simulink model "cukModelStateSpace"  (R2020a)
settings: Solver=FixedStepAuto  StartTime=0.0  StopTime=0.8  RelTol=1e-9  AbsTol=4e-3
undefined symbols (not defined in the file): Asigma, bsigma, Csigma, delta, FaultTypeArray, fdiDevices, fmaxArray, fminArray, Fsigma, Msigma, Nsigma, tfArray, x0, z0
libraries: PhdLibrary x7, powerlib_meascontrol x1
settings Model: SimulationMode=accelerator  Creator=d13go  LastModifiedBy=d13go
settings SolverCC: ZeroCrossControl=DisableAll  ZeroCrossAlgorithm=Adaptive
settings DebuggingCC: IgnoredZcDiagnostic=none

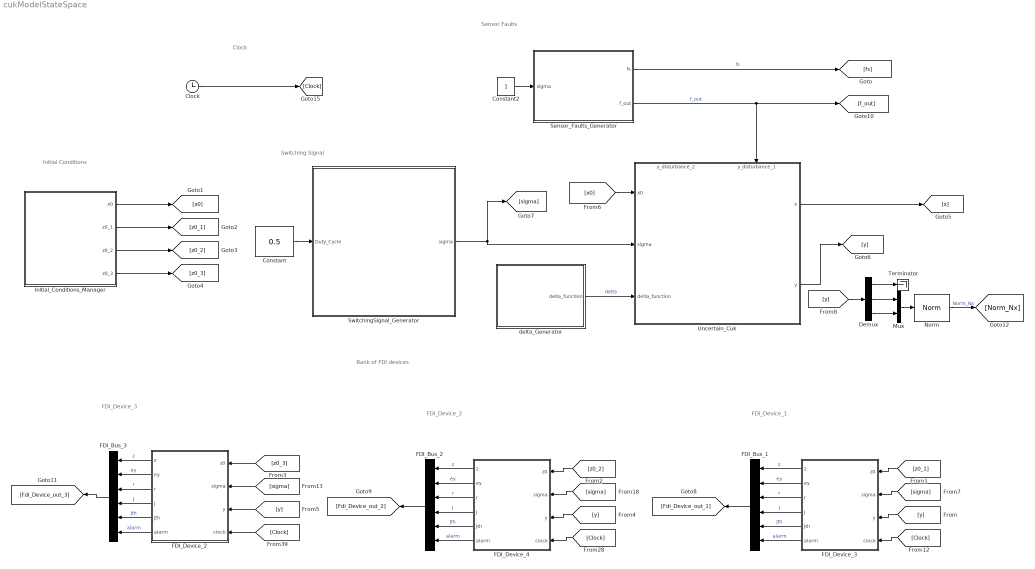
== system cukModelStateSpace ==
  note: Initial Condiitons
  note: Bank of FDI devices
  note: Sensor Faults
  note: FDI_Device_1
  note: FDI_Device_2
  note: FDI_Device_3
  note: Switching Signal
  note: Clock
  Clock : Clock
  Constant : Constant  Value=0.5
  Constant2 : Constant
  Demux : Demux  Outputs=3
  "FDI_Bus_1 " : BusCreator  Inputs=6
  FDI_Bus_2 : BusCreator  Inputs=6
  FDI_Bus_3 : BusCreator  Inputs=6
  FDI_Device_2 : Subsystem  mask{fdiDevice=fdiDevices{3}}
      mask prompts: fdiDevice "FDI Device (Struct)"
      mask Display: fprintf('FDI Device \n Two subsystems');
  FDI_Device_3 : Subsystem  mask{fdiDevice=fdiDevices{1}}
      mask prompts: fdiDevice "FDI Device (Struct)"
      mask Display: fprintf('FDI Device \n Two subsystems');
  FDI_Device_4 : Subsystem  mask{fdiDevice=fdiDevices{2}}
      mask prompts: fdiDevice "FDI Device (Struct)"
      mask Display: fprintf('FDI Device \n Two subsystems');
  Initial_Conditions_Manager : Subsystem
  Mux : Mux  Inputs=2
  Norm : PhdLibrary/Norms/Norm
      settings: SourceProductName=Phd Diego
  Sensor_Faults_Generator : Subsystem
  SwitchingSignal_Generator : Subsystem
  Terminator : Terminator
  Uncertain_Cuk : Subsystem
      settings: PortSchema="{\"entries\":[{\"content\":{\"sides\":[{\"content\":{\"connectorIds\":[\"In1\",\"In2\",\"In3\"]},\"type\":\"ConnectorPlacement.EquallySpacedRectSide\",\"uuid\":\"603634da-9cb1-4386-a493-85de7a0b3601\"},{\"content\":{\"connectorIds\":[\"Out1\",\"Out2\"],\"side\":\"RIGHT\"},\"type\":\"ConnectorPlacement.EquallySpacedRectSide\",\"uuid\":\"04120757-a7c7-4ef9-83e5-a164762aa976\"},{\"content\":{\"connectorIds\":[\"In4\",\"In5\"],\"side\":\"TOP\"},\"type\":\"ConnectorPlacement.EquallySpacedRectSide\",\"uuid\":\"e5c3024c-3e8e-4670-bb80-bfeaf8b64197\"}]},\"type\":\"ConnectorPlacement.EquallySpacedConnector\",\"uuid\":\"63699195-fae3-40a4-a348-448298818555\"}],\"packageUris\":[\"http://schema.mathworks.com/mf0/Connector/19700101\"],\"version\":\"1.0\"}"
  delta_Generator : Subsystem
  wires:
  Clock/1 -> [Clock]
  Sensor_Faults_Generator/2(f_out) -> Uncertain_Cuk/5(y_disturbance_1), [f_out]  "f_out"
  Constant2/1 -> Sensor_Faults_Generator/1(sigma)
  Sensor_Faults_Generator/1(fs) -> [fs]  "fs"
  Initial_Conditions_Manager/1(x0) -> [x0]
  Initial_Conditions_Manager/2(z0_1) -> [z0_1]
  Initial_Conditions_Manager/4(z0_3) -> [z0_3]
  Initial_Conditions_Manager/3(z0_2) -> [z0_2]
  [y] -> FDI_Device_3/3(y)
  [y] -> FDI_Device_4/3(y)
  [y] -> FDI_Device_2/3(y)
  SwitchingSignal_Generator/1(sigma) -> Uncertain_Cuk/2(sigma), [sigma]
  [sigma] -> FDI_Device_3/2(sigma)
  [sigma] -> FDI_Device_4/2(sigma)
  [sigma] -> FDI_Device_2/2(sigma)
  [Clock] -> FDI_Device_3/4(clock)
  [Clock] -> FDI_Device_4/4(clock)
  [Clock] -> FDI_Device_2/4(clock)
  [z0_2] -> FDI_Device_4/1(z0)
  [z0_3] -> FDI_Device_2/1(z0)
  delta_Generator/1(delta_function) -> Uncertain_Cuk/3(delta_function)  "delta"
  Constant/1 -> SwitchingSignal_Generator/1(Duty_Cycle)
  FDI_Device_3/1(z) -> "FDI_Bus_1 "/1  "z"
  FDI_Device_3/2(ey) -> "FDI_Bus_1 "/2  "ey"
  FDI_Device_3/3(r) -> "FDI_Bus_1 "/3  "r"
  FDI_Device_3/4(J) -> "FDI_Bus_1 "/4  "J"
  FDI_Device_4/1(z) -> FDI_Bus_2/1  "z"
  FDI_Device_4/2(ey) -> FDI_Bus_2/2  "ey"
  FDI_Device_4/3(r) -> FDI_Bus_2/3  "r"
  FDI_Device_4/4(J) -> FDI_Bus_2/4  "J"
  FDI_Device_2/1(z) -> FDI_Bus_3/1  "z"
  FDI_Device_2/2(ey) -> FDI_Bus_3/2  "ey"
  FDI_Device_2/3(r) -> FDI_Bus_3/3  "r"
  FDI_Device_2/4(J) -> FDI_Bus_3/4  "J"
  "FDI_Bus_1 "/1 -> [Fdi_Device_out_1]
  FDI_Bus_2/1 -> [Fdi_Device_out_2]
  FDI_Bus_3/1 -> [Fdi_Device_out_3]
  [z0_1] -> FDI_Device_3/1(z0)
  FDI_Device_3/5(Jth) -> "FDI_Bus_1 "/5  "Jth"
  FDI_Device_3/6(alarm) -> "FDI_Bus_1 "/6  "alarm"
  FDI_Device_4/5(Jth) -> FDI_Bus_2/5  "Jth"
  FDI_Device_4/6(alarm) -> FDI_Bus_2/6  "alarm"
  FDI_Device_2/5(Jth) -> FDI_Bus_3/5  "Jth"
  FDI_Device_2/6(alarm) -> FDI_Bus_3/6  "alarm"
  [x0] -> Uncertain_Cuk/1(x0)
  Uncertain_Cuk/2(y) -> [y]
  Uncertain_Cuk/1(x) -> [x]
  ? -> Uncertain_Cuk/4(y_disturbance_2)
  [y] -> Demux/1
  Demux/1 -> Terminator/1
  Mux/1 -> Norm/1
  Norm/1 -> [Norm_Nx]  "Norm_Nx"
  Demux/2 -> Mux/1
  Demux/3 -> Mux/2

== system cukModelStateSpace/FDI_Device_2 ==
  z0 : Inport  PortDimensions=4
  sigma : Inport  Port=2
  y : Inport  Port=3  PortDimensions=3
  clock : Inport  Port=4
  Alarm_Function : Subsystem
  Constant : Constant  Value=fdiDevice.Jth
  Resiual_Evaluation_Function : Subsystem
  Switched Residual Generator2 : Subsystem  AncestorBlock=PhdLibrary/Observers/Switched Residual Generator  mask(Boots State-Space model){reg_z=fdiDevice.regs_z}
      mask prompts: reg_z "Residual error generator (struct)"
      mask help: Boots State-Space model
      mask DialogControl DescTextVar Prompt: dxhat/dt = A(sigma)*xhat+B(sigma)*u + L(sigma)*(y-yhat)
      mask DialogControl Control2 Prompt: yhat = C(sigma)*xhat
      mask DialogControl Control3 Prompt: r = R(sigma)*(y-yhat)
      mask DialogControl Subsystem1 Prompt: Subsystem 1
      mask Display: disp('Switched Luenberger \n Residual Generator \n 2-Subsystems')
  Terminator : Terminator
  z : Outport
  ey : Outport  Port=2
  r : Outport  Port=3
  J : Outport  Port=4
  Jth : Outport  Port=5
  alarm : Outport  Port=6
  wires:
  sigma/1 -> Switched Residual Generator2/2(sigma)
  Alarm_Function/1(alarm) -> alarm/1
  Switched Residual Generator2/4(ey) -> ey/1
  [r] -> r/1
  clock/1 -> [clock]
  [clock] -> Resiual_Evaluation_Function/2(clock)
  Resiual_Evaluation_Function/1(J) -> J/1, Alarm_Function/1(J)
  Switched Residual Generator2/3(r) -> [r], Resiual_Evaluation_Function/1(r)
  Constant/1 -> Jth/1, Alarm_Function/2(Jth)
  y/1 -> Switched Residual Generator2/3(y)
  Switched Residual Generator2/1(z) -> z/1
  z0/1 -> Switched Residual Generator2/1(x0)
  Switched Residual Generator2/2(yhat) -> Terminator/1

== system cukModelStateSpace/FDI_Device_3 ==
  z0 : Inport  PortDimensions=4
  sigma : Inport  Port=2
  y : Inport  Port=3  PortDimensions=3
  clock : Inport  Port=4
  Alarm_Function : Subsystem
  Constant : Constant  Value=fdiDevice.Jth
  Resiual_Evaluation_Function : Subsystem
  Switched Residual Generator2 : Subsystem  AncestorBlock=PhdLibrary/Observers/Switched Residual Generator  mask(Boots State-Space model){reg_z=fdiDevice.regs_z}
      mask prompts: reg_z "Residual error generator (struct)"
      mask help: Boots State-Space model
      mask DialogControl DescTextVar Prompt: dxhat/dt = A(sigma)*xhat+B(sigma)*u + L(sigma)*(y-yhat)
      mask DialogControl Control2 Prompt: yhat = C(sigma)*xhat
      mask DialogControl Control3 Prompt: r = R(sigma)*(y-yhat)
      mask DialogControl Subsystem1 Prompt: Subsystem 1
      mask Display: disp('Switched Luenberger \n Residual Generator \n 2-Subsystems')
  Terminator : Terminator
  z : Outport
  ey : Outport  Port=2
  r : Outport  Port=3
  J : Outport  Port=4
  Jth : Outport  Port=5
  alarm : Outport  Port=6
  wires:
  sigma/1 -> Switched Residual Generator2/2(sigma)
  Alarm_Function/1(alarm) -> alarm/1
  Switched Residual Generator2/4(ey) -> ey/1
  [r] -> r/1
  clock/1 -> [clock]
  [clock] -> Resiual_Evaluation_Function/2(clock)
  Resiual_Evaluation_Function/1(J) -> J/1, Alarm_Function/1(J)
  Switched Residual Generator2/3(r) -> [r], Resiual_Evaluation_Function/1(r)
  Constant/1 -> Jth/1, Alarm_Function/2(Jth)
  y/1 -> Switched Residual Generator2/3(y)
  Switched Residual Generator2/1(z) -> z/1
  z0/1 -> Switched Residual Generator2/1(x0)
  Switched Residual Generator2/2(yhat) -> Terminator/1

== system cukModelStateSpace/FDI_Device_4 ==
  z0 : Inport  PortDimensions=4
  sigma : Inport  Port=2
  y : Inport  Port=3  PortDimensions=3
  clock : Inport  Port=4
  Alarm_Function : Subsystem
  Constant : Constant  Value=fdiDevice.Jth
  Resiual_Evaluation_Function1 : Subsystem
  Switched Residual Generator2 : Subsystem  AncestorBlock=PhdLibrary/Observers/Switched Residual Generator  mask(Boots State-Space model){reg_z=fdiDevice.regs_z}
      mask prompts: reg_z "Residual error generator (struct)"
      mask help: Boots State-Space model
      mask DialogControl DescTextVar Prompt: dxhat/dt = A(sigma)*xhat+B(sigma)*u + L(sigma)*(y-yhat)
      mask DialogControl Control2 Prompt: yhat = C(sigma)*xhat
      mask DialogControl Control3 Prompt: r = R(sigma)*(y-yhat)
      mask DialogControl Subsystem1 Prompt: Subsystem 1
      mask Display: disp('Switched Luenberger \n Residual Generator \n 2-Subsystems')
  Terminator : Terminator
  z : Outport
  ey : Outport  Port=2
  r : Outport  Port=3
  J : Outport  Port=4
  Jth : Outport  Port=5
  alarm : Outport  Port=6
  wires:
  sigma/1 -> Switched Residual Generator2/2(sigma)
  Alarm_Function/1(alarm) -> alarm/1
  Switched Residual Generator2/4(ey) -> ey/1
  [r] -> r/1
  clock/1 -> [clock]
  [clock] -> Resiual_Evaluation_Function1/2(clock)
  Resiual_Evaluation_Function1/1(J) -> J/1, Alarm_Function/1(J)
  Switched Residual Generator2/3(r) -> Resiual_Evaluation_Function1/1(r), [r]
  Constant/1 -> Jth/1, Alarm_Function/2(Jth)
  y/1 -> Switched Residual Generator2/3(y)
  Switched Residual Generator2/1(z) -> z/1
  z0/1 -> Switched Residual Generator2/1(x0)
  Switched Residual Generator2/2(yhat) -> Terminator/1

== system cukModelStateSpace/Initial_Conditions_Manager ==
  Ground1 : Ground
  IC1 : InitialCondition  Value=[x0]
  IC2 : InitialCondition  Value=[z0]
  Mux2 : Mux
  x0 : Outport
  z0_1 : Outport  Port=2
  z0_2 : Outport  Port=3
  z0_3 : Outport  Port=4
  wires:
  Mux2/1 -> IC1/1, IC2/1
  Ground1/1 -> Mux2/3, Mux2/4, Mux2/2, Mux2/1
  IC1/1 -> z0_1/1, x0/1
  IC2/1 -> z0_3/1, z0_2/1

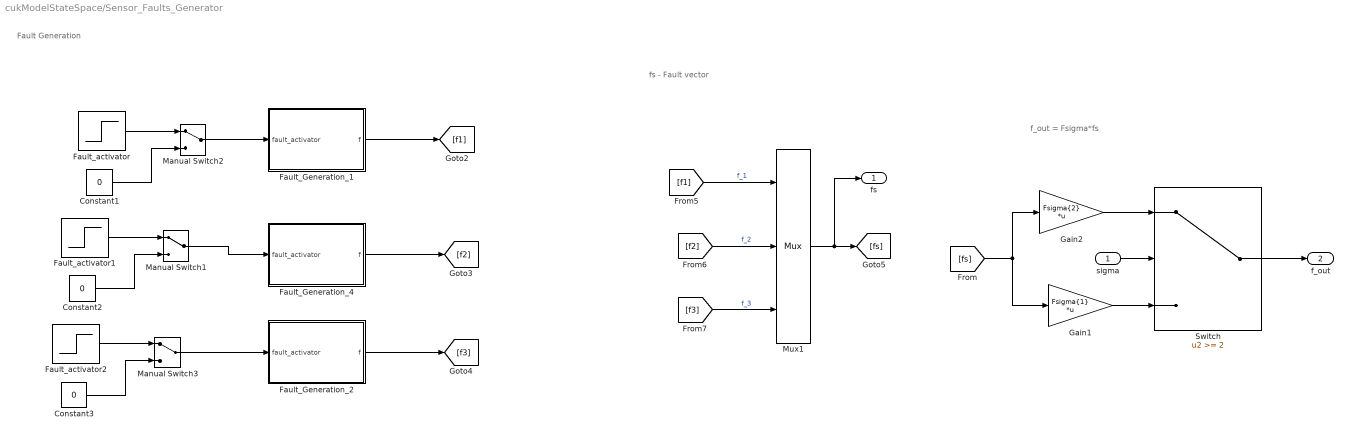
== system cukModelStateSpace/Sensor_Faults_Generator ==
  note: fs - Fault vector
  note: Fault Generation
  note: f_out = Fsigma*fs
  sigma : Inport
  Constant1 : Constant  Value=0
  Constant2 : Constant  Value=0
  Constant3 : Constant  Value=0
  Fault_Generation_1 : Subsystem  mask{fmax=fmaxArray(1), fmin=fminArray(1)}
      mask prompts: fmax "Maximum magnitude of the fault"; fmin "Minimum magnitude of the fault"
      mask DialogControl DescTextVar Prompt: Offset fatul generator.
      mask DialogControl DescTextVar_copy Prompt: Fault_activator:  0: f = 0; 1: f = fmax;  2  f =fmin
      mask Display: fprintf('Offset fault generator \n with two levels')
  Fault_Generation_2 : Subsystem  mask{fmax=fmaxArray(3), fmin=fminArray(3)}
      mask prompts: fmax "Maximum magnitude of the fault"; fmin "Minimum magnitude of the fault"
      mask DialogControl DescTextVar Prompt: Offset fatul generator.
      mask DialogControl DescTextVar_copy Prompt: Fault_activator:  0: f = 0; 1: f = fmax;  2  f =fmin
      mask Display: fprintf('Offset fault generator \n with two levels')
  Fault_Generation_4 : Subsystem  mask{fmax=fmaxArray(2), fmin=fminArray(2)}
      mask prompts: fmax "Maximum magnitude of the fault"; fmin "Minimum magnitude of the fault"
      mask DialogControl DescTextVar Prompt: Offset fatul generator.
      mask DialogControl DescTextVar_copy Prompt: Fault_activator:  0: f = 0; 1: f = fmax;  2  f =fmin
      mask Display: fprintf('Offset fault generator \n with two levels')
  Fault_activator : Step  Time=tfArray(1)  After=FaultTypeArray(1)  SampleTime=0
  Fault_activator1 : Step  Time=tfArray(2)  After=FaultTypeArray(2)  SampleTime=0
  Fault_activator2 : Step  Time=tfArray(3)  After=FaultTypeArray(3)  SampleTime=0
  Gain1 : Gain  Gain=Fsigma{1}  Multiplication=Matrix(K*u) (u vector)
  Gain2 : Gain  Gain=Fsigma{2}  Multiplication=Matrix(K*u) (u vector)
  Manual Switch1 : ManualSwitch
  Manual Switch2 : ManualSwitch
  Manual Switch3 : ManualSwitch
  Mux1 : Mux  Inputs=3
      settings: DisplayOption=signals
  Switch : Switch  Threshold=2
  fs : Outport
  f_out : Outport  Port=2
  wires:
  Fault_Generation_4/1(f) -> [f2]
  [f1] -> Mux1/1  "f_1"
  [f2] -> Mux1/2  "f_2"
  [f3] -> Mux1/3  "f_3"
  Mux1/1 -> fs/1, [fs]
  sigma/1 -> Switch/2
  Gain1/1 -> Switch/3
  [fs] -> Gain2/1, Gain1/1
  Fault_Generation_1/1(f) -> [f1]
  Constant1/1 -> Manual Switch2/2
  Fault_activator/1 -> Manual Switch2/1
  Manual Switch2/1 -> Fault_Generation_1/1(fault_activator)
  Manual Switch1/1 -> Fault_Generation_4/1(fault_activator)
  Fault_activator1/1 -> Manual Switch1/1
  Constant2/1 -> Manual Switch1/2
  Manual Switch3/1 -> Fault_Generation_2/1(fault_activator)
  Fault_activator2/1 -> Manual Switch3/1
  Constant3/1 -> Manual Switch3/2
  Fault_Generation_2/1(f) -> [f3]
  Switch/1 -> f_out/1
  Gain2/1 -> Switch/1

== system cukModelStateSpace/SwitchingSignal_Generator ==
  Duty_Cycle : Inport
  Constant : Constant  Value=2
  PWM Generator (DC-DC)1 : powerlib_meascontrol/Pulse & Signal Generators/PWM Generator (DC-DC)  Fsw=20000  Ts=0
  Sum : Sum  Inputs=|-+
  sigma : Outport
  wires:
  Duty_Cycle/1 -> PWM Generator (DC-DC)1/1
  Constant/1 -> Sum/2
  PWM Generator (DC-DC)1/1 -> Sum/1
  Sum/1 -> sigma/1

== system cukModelStateSpace/Uncertain_Cuk ==
  x0 : Inport  PortDimensions=4
  sigma : Inport  Port=2
  delta_function : Inport  Port=3
  y_disturbance_2 : Inport  Port=4  PortDimensions=3
  y_disturbance_1 : Inport  Port=5  PortDimensions=3
  Uncertain Cuk : Subsystem  mask{A1=Asigma{1}, B1=bsigma{1}, C1=Csigma{1}, A2=Asigma{2}, B2=bsigma{2}, C2=Csigma{2}}
      mask prompts: A1 "Matrix A"; B1 "Matrix B"; C1 "Matrix C"; A2 "Matrix A"; B2 "Matrix B"; C2 "Matrix C"
      mask DialogControl DescTextVar Prompt: dx/dt = A(sigma)x+ b(sigma) + wx(sigma,x,u,t)
      mask DialogControl Control2 Prompt: y = C(sigma)x + wy(sigma,x,u,t)
      mask DialogControl Container3 Prompt: Subsystem 1
      mask DialogControl Container4 Prompt: Subsystem 2
      mask Display: disp('Switched Affine System State Space  \n with perturbations \n 2-Subsystems')
  Uncertainty_System_1 : Subsystem  mask{M=Msigma{1}, N=Nsigma{1}}
      mask prompts: M "M matrix"; N "N matrix"
      mask DialogControl DescTextVar Prompt: Uncertainties matrices of type \DeltaA = delta(t)*MaNa*x(t)
      mask Display: disp('Norm-bounded \n uncertainty')
  Uncertainty_System_2 : Subsystem  mask{M=Msigma{2}, N=Nsigma{2}}
      mask prompts: M "M matrix"; N "N matrix"
      mask DialogControl DescTextVar Prompt: Uncertainties matrices of type \DeltaA = delta(t)*MaNa*x(t)
      mask Display: disp('Norm-bounded \n uncertainty')
  x : Outport
  y : Outport  Port=2
  wires:
  [x] -> Uncertainty_System_2/2(x), Uncertainty_System_1/2(x)
  Uncertainty_System_2/1(DeltaAx) -> [DeltaA2x]
  Uncertain Cuk/1(x) -> x/1, [x]
  Uncertain Cuk/2(y) -> y/1
  delta_function/1 -> Uncertainty_System_1/1(delta_function), Uncertainty_System_2/1(delta_function)
  sigma/1 -> Uncertain Cuk/2(sigma)
  x0/1 -> Uncertain Cuk/1(x0)
  [DeltaA2x] -> Uncertain Cuk/5(x_disturbance_2)
  [DeltaA1x] -> Uncertain Cuk/3(x_disturbance_1)
  y_disturbance_2/1 -> Uncertain Cuk/6(y_disturbance_2)
  y_disturbance_1/1 -> Uncertain Cuk/4(y_disturbance_1)
  Uncertainty_System_1/1(DeltaAx) -> [DeltaA1x]

== system cukModelStateSpace/delta_Generator ==
  Constant : Constant  Value=0
  Manual Switch : ManualSwitch
  Sinusoidal : SignalGenerator  Amplitude=delta  Frequency=60  Units=rad/sec
  delta_function : Outport
  wires:
  Sinusoidal/1 -> Manual Switch/1
  Manual Switch/1 -> [delta], delta_function/1
  Constant/1 -> Manual Switch/2

== system cukModelStateSpace/FDI_Device_2/Alarm_Function ==
  note: If J(r)>=Jth, then a fault has occurred
  J : Inport
  Jth : Inport  Port=2
  Cast To Double : DataTypeConversion  OutDataTypeStr=double
  Constant : Constant
  Constant1 : Constant  Value=0
  GreaterThan : RelationalOperator  OutDataTypeStr=boolean  RndMeth=Simplest
  If : If
  If Action Subsystem : Subsystem  TreatAsAtomicUnit=on
  If Action Subsystem1 : Subsystem  TreatAsAtomicUnit=on
  Merge : Merge
  alarm : Outport
  wires:
  J/1 -> GreaterThan/1
  Jth/1 -> GreaterThan/2
  If/1 -> If Action Subsystem/Action
  Constant/1 -> If Action Subsystem/1(In1)
  If/2 -> If Action Subsystem1/Action
  Constant1/1 -> If Action Subsystem1/1(In1)
  If Action Subsystem/1(Out1) -> Merge/1
  If Action Subsystem1/1(Out1) -> Merge/2
  Merge/1 -> alarm/1
  GreaterThan/1 -> Cast To Double/1
  Cast To Double/1 -> If/1

== system cukModelStateSpace/FDI_Device_2/Resiual_Evaluation_Function ==
  r : Inport
  clock : Inport  Port=2
  Delay : Delay  DelayLength=1  SampleTime=fdiDevice.T
  If : If  IfExpression=u1 >= T
  If Action Subsystem : Subsystem  TreatAsAtomicUnit=on
  If Action Subsystem1 : Subsystem  TreatAsAtomicUnit=on
  Max : MinMax  Function=max  Inputs=2
  Merge : Merge
  Norm3 : PhdLibrary/Norms/Norm
      settings: SourceProductName=Phd Diego
  J : Outport
  wires:
  clock/1 -> If/1
  If/1 -> If Action Subsystem/Action
  If/2 -> If Action Subsystem1/Action
  r/1 -> [r]
  [r] -> Norm3/1
  [r] -> If Action Subsystem1/1(r)
  If Action Subsystem/1(J) -> Merge/1
  If Action Subsystem1/1(J) -> Merge/2
  Merge/1 -> J/1
  Delay/1 -> Max/2
  Norm3/1 -> Max/1, Delay/1  "||r1||"
  Max/1 -> If Action Subsystem/1(r)

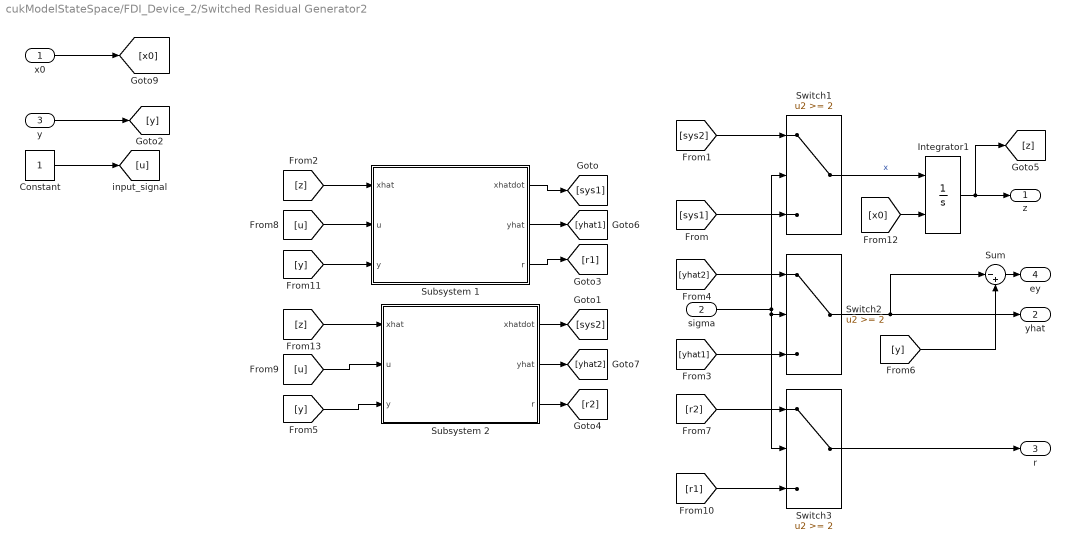
== system cukModelStateSpace/FDI_Device_2/Switched Residual Generator2 ==
  x0 : Inport
  sigma : Inport  Port=2
  y : Inport  Port=3
  Constant : Constant
  Integrator1 : Integrator  InitialConditionSource=external  InitialCondition=[0; 0; 0;0]
  Subsystem 1 : Subsystem  mask{A=reg_z.Asigma{1}, B=reg_z.bsigma{1}, L=reg_z.Lsigma{1}, C=reg_z.Csigma{1}, R=reg_z.Rsigma{1}}
      mask prompts: A "Matrix A"; B "Matrix B"; L "Matrix L"; C "Matrix C"; R "Matrix R"
      mask DialogControl DescTextVar Prompt: dxhat/dt = A*xhat + B*u + L*(y-yhat)
      mask DialogControl Control2 Prompt: yhat = C*xhat
      mask Display: disp('Luenberger Residual \n Generator')
  Subsystem 2 : Subsystem  mask{A=reg_z.Asigma{2}, B=reg_z.bsigma{2}, L=reg_z.Lsigma{2}, C=reg_z.Csigma{2}, R=reg_z.Rsigma{2}}
      mask prompts: A "Matrix A"; B "Matrix B"; L "Matrix L"; C "Matrix C"; R "Matrix R"
      mask DialogControl DescTextVar Prompt: dxhat/dt = A*xhat + B*u + L*(y-yhat)
      mask DialogControl Control2 Prompt: yhat = C*xhat
      mask Display: disp('Luenberger Residual \n Generator')
  Sum : Sum  Inputs=|-+
  Switch1 : Switch  Threshold=2
  Switch2 : Switch  Threshold=2
  Switch3 : Switch  Threshold=2
  z : Outport
  yhat : Outport  Port=2
  r : Outport  Port=3
  ey : Outport  Port=4
  wires:
  [yhat2] -> Switch2/1
  [yhat1] -> Switch2/3
  [y] -> Sum/2
  Sum/1 -> ey/1
  y/1 -> [y]
  [y] -> Subsystem 2/3(y)
  Switch3/1 -> r/1
  Switch2/1 -> yhat/1, Sum/1
  [r1] -> Switch3/3
  [r2] -> Switch3/1
  Subsystem 2/2(yhat) -> [yhat2]
  Subsystem 1/2(yhat) -> [yhat1]
  Subsystem 2/3(r) -> [r2]
  Subsystem 1/3(r) -> [r1]
  Subsystem 2/1(xhatdot) -> [sys2]
  Subsystem 1/1(xhatdot) -> [sys1]
  x0/1 -> [x0]
  Switch1/1 -> Integrator1/1  "x"
  [sys1] -> Switch1/3
  [sys2] -> Switch1/1
  Integrator1/1 -> [z], z/1
  sigma/1 -> Switch1/2, Switch2/2, Switch3/2
  Constant/1 -> [u]
  [u] -> Subsystem 1/2(u)
  [u] -> Subsystem 2/2(u)
  [y] -> Subsystem 1/3(y)
  [z] -> Subsystem 1/1(xhat)
  [z] -> Subsystem 2/1(xhat)
  [x0] -> Integrator1/2

== system cukModelStateSpace/FDI_Device_3/Alarm_Function ==
  note: If J(r)>=Jth, then a fault has occurred
  J : Inport
  Jth : Inport  Port=2
  Cast To Double : DataTypeConversion  OutDataTypeStr=double
  Constant : Constant
  Constant1 : Constant  Value=0
  GreaterThan : RelationalOperator  OutDataTypeStr=boolean  RndMeth=Simplest
  If : If
  If Action Subsystem : Subsystem  TreatAsAtomicUnit=on
  If Action Subsystem1 : Subsystem  TreatAsAtomicUnit=on
  Merge : Merge
  alarm : Outport
  wires:
  J/1 -> GreaterThan/1
  Jth/1 -> GreaterThan/2
  If/1 -> If Action Subsystem/Action
  Constant/1 -> If Action Subsystem/1(In1)
  If/2 -> If Action Subsystem1/Action
  Constant1/1 -> If Action Subsystem1/1(In1)
  If Action Subsystem/1(Out1) -> Merge/1
  If Action Subsystem1/1(Out1) -> Merge/2
  Merge/1 -> alarm/1
  GreaterThan/1 -> Cast To Double/1
  Cast To Double/1 -> If/1

== system cukModelStateSpace/FDI_Device_3/Resiual_Evaluation_Function ==
  r : Inport
  clock : Inport  Port=2
  Delay : Delay  DelayLength=1  SampleTime=fdiDevice.T
  If : If  IfExpression=u1 >= T
  If Action Subsystem : Subsystem  TreatAsAtomicUnit=on
  If Action Subsystem1 : Subsystem  TreatAsAtomicUnit=on
  Max : MinMax  Function=max  Inputs=2
  Merge : Merge
  Norm3 : PhdLibrary/Norms/Norm
      settings: SourceProductName=Phd Diego
  J : Outport
  wires:
  clock/1 -> If/1
  If/1 -> If Action Subsystem/Action
  If/2 -> If Action Subsystem1/Action
  r/1 -> [r]
  [r] -> Norm3/1
  [r] -> If Action Subsystem1/1(r)
  If Action Subsystem/1(J) -> Merge/1
  If Action Subsystem1/1(J) -> Merge/2
  Merge/1 -> J/1
  Delay/1 -> Max/2
  Norm3/1 -> Max/1, Delay/1  "||r1||"
  Max/1 -> If Action Subsystem/1(r)

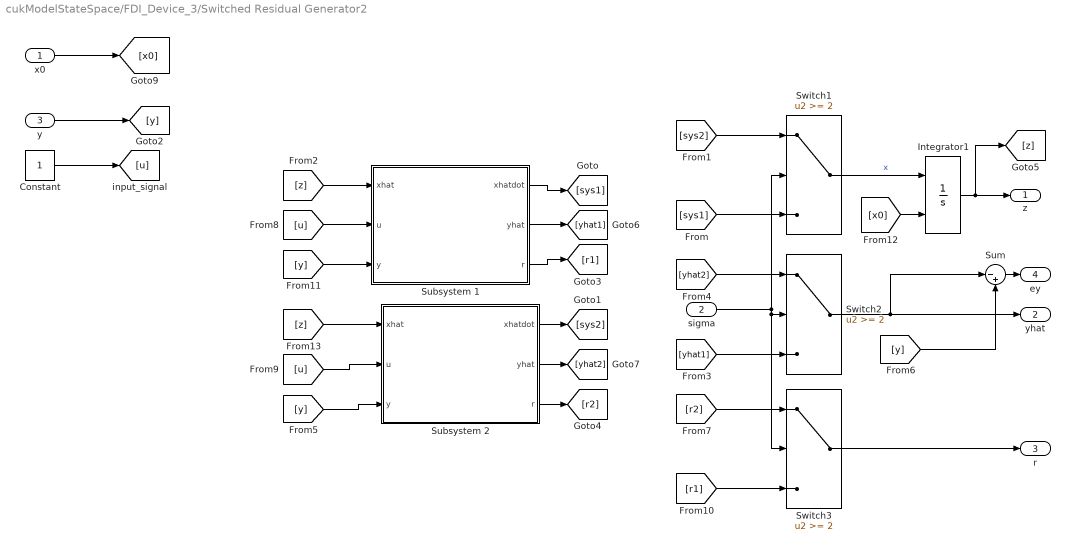
== system cukModelStateSpace/FDI_Device_3/Switched Residual Generator2 ==
  x0 : Inport
  sigma : Inport  Port=2
  y : Inport  Port=3
  Constant : Constant
  Integrator1 : Integrator  InitialConditionSource=external  InitialCondition=[0; 0; 0;0]
  Subsystem 1 : Subsystem  mask{A=reg_z.Asigma{1}, B=reg_z.bsigma{1}, L=reg_z.Lsigma{1}, C=reg_z.Csigma{1}, R=reg_z.Rsigma{1}}
      mask prompts: A "Matrix A"; B "Matrix B"; L "Matrix L"; C "Matrix C"; R "Matrix R"
      mask DialogControl DescTextVar Prompt: dxhat/dt = A*xhat + B*u + L*(y-yhat)
      mask DialogControl Control2 Prompt: yhat = C*xhat
      mask Display: disp('Luenberger Residual \n Generator')
  Subsystem 2 : Subsystem  mask{A=reg_z.Asigma{2}, B=reg_z.bsigma{2}, L=reg_z.Lsigma{2}, C=reg_z.Csigma{2}, R=reg_z.Rsigma{2}}
      mask prompts: A "Matrix A"; B "Matrix B"; L "Matrix L"; C "Matrix C"; R "Matrix R"
      mask DialogControl DescTextVar Prompt: dxhat/dt = A*xhat + B*u + L*(y-yhat)
      mask DialogControl Control2 Prompt: yhat = C*xhat
      mask Display: disp('Luenberger Residual \n Generator')
  Sum : Sum  Inputs=|-+
  Switch1 : Switch  Threshold=2
  Switch2 : Switch  Threshold=2
  Switch3 : Switch  Threshold=2
  z : Outport
  yhat : Outport  Port=2
  r : Outport  Port=3
  ey : Outport  Port=4
  wires:
  [yhat2] -> Switch2/1
  [yhat1] -> Switch2/3
  [y] -> Sum/2
  Sum/1 -> ey/1
  y/1 -> [y]
  [y] -> Subsystem 2/3(y)
  Switch3/1 -> r/1
  Switch2/1 -> yhat/1, Sum/1
  [r1] -> Switch3/3
  [r2] -> Switch3/1
  Subsystem 2/2(yhat) -> [yhat2]
  Subsystem 1/2(yhat) -> [yhat1]
  Subsystem 2/3(r) -> [r2]
  Subsystem 1/3(r) -> [r1]
  Subsystem 2/1(xhatdot) -> [sys2]
  Subsystem 1/1(xhatdot) -> [sys1]
  x0/1 -> [x0]
  Switch1/1 -> Integrator1/1  "x"
  [sys1] -> Switch1/3
  [sys2] -> Switch1/1
  Integrator1/1 -> [z], z/1
  sigma/1 -> Switch1/2, Switch2/2, Switch3/2
  Constant/1 -> [u]
  [u] -> Subsystem 1/2(u)
  [u] -> Subsystem 2/2(u)
  [y] -> Subsystem 1/3(y)
  [z] -> Subsystem 1/1(xhat)
  [z] -> Subsystem 2/1(xhat)
  [x0] -> Integrator1/2

== system cukModelStateSpace/FDI_Device_4/Alarm_Function ==
  note: If J(r)>=Jth, then a fault has occurred
  J : Inport
  Jth : Inport  Port=2
  Cast To Double : DataTypeConversion  OutDataTypeStr=double
  Constant : Constant
  Constant1 : Constant  Value=0
  GreaterThan : RelationalOperator  OutDataTypeStr=boolean  RndMeth=Simplest
  If : If
  If Action Subsystem : Subsystem  TreatAsAtomicUnit=on
  If Action Subsystem1 : Subsystem  TreatAsAtomicUnit=on
  Merge : Merge
  alarm : Outport
  wires:
  J/1 -> GreaterThan/1
  Jth/1 -> GreaterThan/2
  If/1 -> If Action Subsystem/Action
  Constant/1 -> If Action Subsystem/1(In1)
  If/2 -> If Action Subsystem1/Action
  Constant1/1 -> If Action Subsystem1/1(In1)
  If Action Subsystem/1(Out1) -> Merge/1
  If Action Subsystem1/1(Out1) -> Merge/2
  Merge/1 -> alarm/1
  GreaterThan/1 -> Cast To Double/1
  Cast To Double/1 -> If/1

== system cukModelStateSpace/FDI_Device_4/Resiual_Evaluation_Function1 ==
  r : Inport
  clock : Inport  Port=2
  Delay : Delay  DelayLength=1  SampleTime=fdiDevice.T
  If : If  IfExpression=u1 >= T
  If Action Subsystem : Subsystem  TreatAsAtomicUnit=on
  If Action Subsystem1 : Subsystem  TreatAsAtomicUnit=on
  Max : MinMax  Function=max  Inputs=2
  Merge : Merge
  Norm3 : PhdLibrary/Norms/Norm
      settings: SourceProductName=Phd Diego
  J : Outport
  wires:
  clock/1 -> If/1
  If/1 -> If Action Subsystem/Action
  If/2 -> If Action Subsystem1/Action
  r/1 -> [r]
  [r] -> Norm3/1
  [r] -> If Action Subsystem1/1(r)
  If Action Subsystem/1(J) -> Merge/1
  If Action Subsystem1/1(J) -> Merge/2
  Merge/1 -> J/1
  Delay/1 -> Max/2
  Norm3/1 -> Max/1, Delay/1  "||r1||"
  Max/1 -> If Action Subsystem/1(r)

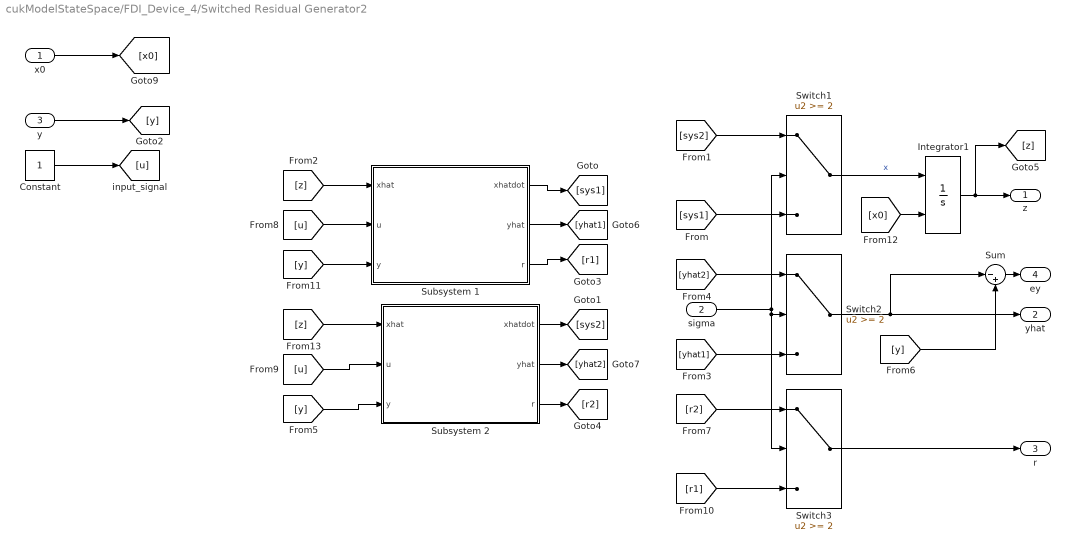
== system cukModelStateSpace/FDI_Device_4/Switched Residual Generator2 ==
  x0 : Inport
  sigma : Inport  Port=2
  y : Inport  Port=3
  Constant : Constant
  Integrator1 : Integrator  InitialConditionSource=external  InitialCondition=[0; 0; 0;0]
  Subsystem 1 : Subsystem  mask{A=reg_z.Asigma{1}, B=reg_z.bsigma{1}, L=reg_z.Lsigma{1}, C=reg_z.Csigma{1}, R=reg_z.Rsigma{1}}
      mask prompts: A "Matrix A"; B "Matrix B"; L "Matrix L"; C "Matrix C"; R "Matrix R"
      mask DialogControl DescTextVar Prompt: dxhat/dt = A*xhat + B*u + L*(y-yhat)
      mask DialogControl Control2 Prompt: yhat = C*xhat
      mask Display: disp('Luenberger Residual \n Generator')
  Subsystem 2 : Subsystem  mask{A=reg_z.Asigma{2}, B=reg_z.bsigma{2}, L=reg_z.Lsigma{2}, C=reg_z.Csigma{2}, R=reg_z.Rsigma{2}}
      mask prompts: A "Matrix A"; B "Matrix B"; L "Matrix L"; C "Matrix C"; R "Matrix R"
      mask DialogControl DescTextVar Prompt: dxhat/dt = A*xhat + B*u + L*(y-yhat)
      mask DialogControl Control2 Prompt: yhat = C*xhat
      mask Display: disp('Luenberger Residual \n Generator')
  Sum : Sum  Inputs=|-+
  Switch1 : Switch  Threshold=2
  Switch2 : Switch  Threshold=2
  Switch3 : Switch  Threshold=2
  z : Outport
  yhat : Outport  Port=2
  r : Outport  Port=3
  ey : Outport  Port=4
  wires:
  [yhat2] -> Switch2/1
  [yhat1] -> Switch2/3
  [y] -> Sum/2
  Sum/1 -> ey/1
  y/1 -> [y]
  [y] -> Subsystem 2/3(y)
  Switch3/1 -> r/1
  Switch2/1 -> yhat/1, Sum/1
  [r1] -> Switch3/3
  [r2] -> Switch3/1
  Subsystem 2/2(yhat) -> [yhat2]
  Subsystem 1/2(yhat) -> [yhat1]
  Subsystem 2/3(r) -> [r2]
  Subsystem 1/3(r) -> [r1]
  Subsystem 2/1(xhatdot) -> [sys2]
  Subsystem 1/1(xhatdot) -> [sys1]
  x0/1 -> [x0]
  Switch1/1 -> Integrator1/1  "x"
  [sys1] -> Switch1/3
  [sys2] -> Switch1/1
  Integrator1/1 -> [z], z/1
  sigma/1 -> Switch1/2, Switch2/2, Switch3/2
  Constant/1 -> [u]
  [u] -> Subsystem 1/2(u)
  [u] -> Subsystem 2/2(u)
  [y] -> Subsystem 1/3(y)
  [z] -> Subsystem 1/1(xhat)
  [z] -> Subsystem 2/1(xhat)
  [x0] -> Integrator1/2

== system cukModelStateSpace/Sensor_Faults_Generator/Fault_Generation_1 ==
  fault_activator : Inport
  Constant1 : Constant  Value=fmin
  Constant2 : Constant  Value=fmax
  Constant3 : Constant  Value=0
  Constant6 : Constant  Value=0
  Merge : Merge  Inputs=4
  Switch Case : SwitchCase  CaseConditions={0,1,2}
  Switch Case Action Subsystem : Subsystem  TreatAsAtomicUnit=on
  Switch Case Action Subsystem1 : Subsystem  TreatAsAtomicUnit=on
  Switch Case Action Subsystem2 : Subsystem  TreatAsAtomicUnit=on
  Switch Case Action Subsystem3 : Subsystem  TreatAsAtomicUnit=on
  f : Outport
  wires:
  Constant2/1 -> Switch Case Action Subsystem/1(In1)
  Constant1/1 -> Switch Case Action Subsystem1/1(In1)
  Constant6/1 -> Switch Case Action Subsystem2/1(In1)
  Constant3/1 -> Switch Case Action Subsystem3/1(In1)
  Switch Case/1 -> Switch Case Action Subsystem3/Action
  Switch Case/2 -> Switch Case Action Subsystem/Action
  Switch Case/3 -> Switch Case Action Subsystem1/Action
  Switch Case/4 -> Switch Case Action Subsystem2/Action
  Switch Case Action Subsystem3/1(Out1) -> Merge/1
  Switch Case Action Subsystem/1(Out1) -> Merge/2
  Switch Case Action Subsystem1/1(Out1) -> Merge/3
  Switch Case Action Subsystem2/1(Out1) -> Merge/4
  Merge/1 -> f/1
  fault_activator/1 -> Switch Case/1

== system cukModelStateSpace/Sensor_Faults_Generator/Fault_Generation_2 ==
  fault_activator : Inport
  Constant1 : Constant  Value=fmin
  Constant2 : Constant  Value=fmax
  Constant3 : Constant  Value=0
  Constant6 : Constant  Value=0
  Merge : Merge  Inputs=4
  Switch Case : SwitchCase  CaseConditions={0,1,2}
  Switch Case Action Subsystem : Subsystem  TreatAsAtomicUnit=on
  Switch Case Action Subsystem1 : Subsystem  TreatAsAtomicUnit=on
  Switch Case Action Subsystem2 : Subsystem  TreatAsAtomicUnit=on
  Switch Case Action Subsystem3 : Subsystem  TreatAsAtomicUnit=on
  f : Outport
  wires:
  Constant2/1 -> Switch Case Action Subsystem/1(In1)
  Constant1/1 -> Switch Case Action Subsystem1/1(In1)
  Constant6/1 -> Switch Case Action Subsystem2/1(In1)
  Constant3/1 -> Switch Case Action Subsystem3/1(In1)
  Switch Case/1 -> Switch Case Action Subsystem3/Action
  Switch Case/2 -> Switch Case Action Subsystem/Action
  Switch Case/3 -> Switch Case Action Subsystem1/Action
  Switch Case/4 -> Switch Case Action Subsystem2/Action
  Switch Case Action Subsystem3/1(Out1) -> Merge/1
  Switch Case Action Subsystem/1(Out1) -> Merge/2
  Switch Case Action Subsystem1/1(Out1) -> Merge/3
  Switch Case Action Subsystem2/1(Out1) -> Merge/4
  Merge/1 -> f/1
  fault_activator/1 -> Switch Case/1

== system cukModelStateSpace/Sensor_Faults_Generator/Fault_Generation_4 ==
  fault_activator : Inport
  Constant1 : Constant  Value=fmin
  Constant2 : Constant  Value=fmax
  Constant3 : Constant  Value=0
  Constant6 : Constant  Value=0
  Merge : Merge  Inputs=4
  Switch Case : SwitchCase  CaseConditions={0,1,2}
  Switch Case Action Subsystem : Subsystem  TreatAsAtomicUnit=on
  Switch Case Action Subsystem1 : Subsystem  TreatAsAtomicUnit=on
  Switch Case Action Subsystem2 : Subsystem  TreatAsAtomicUnit=on
  Switch Case Action Subsystem3 : Subsystem  TreatAsAtomicUnit=on
  f : Outport
  wires:
  Constant2/1 -> Switch Case Action Subsystem/1(In1)
  Constant1/1 -> Switch Case Action Subsystem1/1(In1)
  Constant6/1 -> Switch Case Action Subsystem2/1(In1)
  Constant3/1 -> Switch Case Action Subsystem3/1(In1)
  Switch Case/1 -> Switch Case Action Subsystem3/Action
  Switch Case/2 -> Switch Case Action Subsystem/Action
  Switch Case/3 -> Switch Case Action Subsystem1/Action
  Switch Case/4 -> Switch Case Action Subsystem2/Action
  Switch Case Action Subsystem3/1(Out1) -> Merge/1
  Switch Case Action Subsystem/1(Out1) -> Merge/2
  Switch Case Action Subsystem1/1(Out1) -> Merge/3
  Switch Case Action Subsystem2/1(Out1) -> Merge/4
  Merge/1 -> f/1
  fault_activator/1 -> Switch Case/1

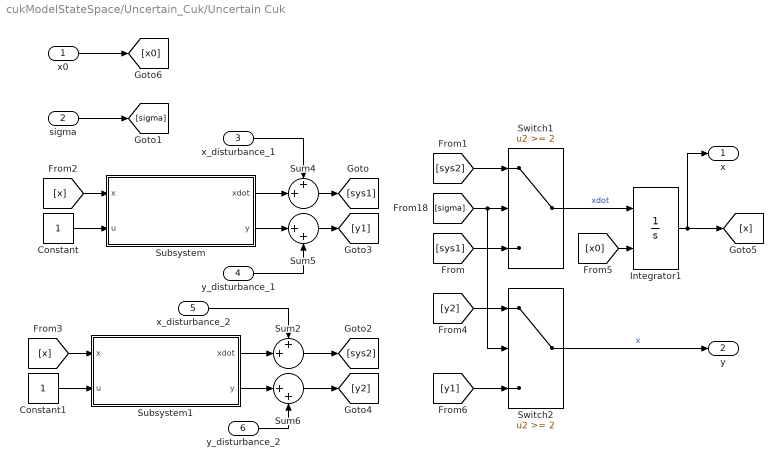
== system cukModelStateSpace/Uncertain_Cuk/Uncertain Cuk ==
  x0 : Inport
  sigma : Inport  Port=2
  x_disturbance_1 : Inport  Port=3
  y_disturbance_1 : Inport  Port=4
  x_disturbance_2 : Inport  Port=5
  y_disturbance_2 : Inport  Port=6
  Constant : Constant
  Constant1 : Constant
  Integrator1 : Integrator  InitialConditionSource=external  InitialCondition=[0;0; 0; 0]
  Subsystem : Subsystem  mask{A=A1, B=B1, C=C1}
      mask prompts: A "Matrix A"; B "Matrix B"; C "Matrix C"
      mask Display: disp('Static State Space \n xdot = Ax+Bu\n y =Cx')
  Subsystem1 : Subsystem  mask{A=A2, B=B2, C=C2}
      mask prompts: A "Matrix A"; B "Matrix B"; C "Matrix C"
      mask Display: disp('Static State Space \n xdot = Ax+Bu\n y =Cx')
  Sum2 : Sum  Inputs=++|
  Sum4 : Sum  Inputs=++|
  Sum5 : Sum  Inputs=|++
  Sum6 : Sum  Inputs=|++
  Switch1 : Switch  Threshold=2
  Switch2 : Switch  Threshold=2
  x : Outport
  y : Outport  Port=2
  wires:
  [sys2] -> Switch1/1
  [sys1] -> Switch1/3
  [sigma] -> Switch2/2, Switch1/2
  Subsystem/1(xdot) -> Sum4/2
  Subsystem/2(y) -> Sum5/1
  Sum4/1 -> [sys1]
  Sum5/1 -> [y1]
  [x] -> Subsystem/1(x)
  Constant/1 -> Subsystem/2(u)
  Switch1/1 -> Integrator1/1  "xdot"
  [x0] -> Integrator1/2
  Integrator1/1 -> x/1, [x]
  Sum6/1 -> [y2]
  Sum2/1 -> [sys2]
  Subsystem1/2(y) -> Sum6/1
  [x] -> Subsystem1/1(x)
  Subsystem1/1(xdot) -> Sum2/2
  Constant1/1 -> Subsystem1/2(u)
  [y2] -> Switch2/1
  [y1] -> Switch2/3
  Switch2/1 -> y/1  "x"
  sigma/1 -> [sigma]
  x0/1 -> [x0]
  x_disturbance_1/1 -> Sum4/1
  y_disturbance_1/1 -> Sum5/2
  x_disturbance_2/1 -> Sum2/1
  y_disturbance_2/1 -> Sum6/2

== system cukModelStateSpace/Uncertain_Cuk/Uncertainty_System_1 ==
  delta_function : Inport
  x : Inport  Port=2
  Constant : Constant  Value=M
  Constant1 : Constant  Value=N
  Matrix Multiply1 : Product
  Matrix Multiply2 : Product  Multiplication=Matrix(*)
  Matrix Multiply3 : Product  Multiplication=Matrix(*)
  DeltaAx : Outport
  wires:
  Constant/1 -> Matrix Multiply3/1
  Constant1/1 -> Matrix Multiply3/2
  Matrix Multiply3/1 -> Matrix Multiply1/2
  delta_function/1 -> Matrix Multiply1/1
  Matrix Multiply1/1 -> Matrix Multiply2/1
  x/1 -> Matrix Multiply2/2
  Matrix Multiply2/1 -> DeltaAx/1

== system cukModelStateSpace/Uncertain_Cuk/Uncertainty_System_2 ==
  delta_function : Inport
  x : Inport  Port=2
  Constant : Constant  Value=M
  Constant1 : Constant  Value=N
  Matrix Multiply1 : Product
  Matrix Multiply2 : Product  Multiplication=Matrix(*)
  Matrix Multiply3 : Product  Multiplication=Matrix(*)
  DeltaAx : Outport
  wires:
  Constant/1 -> Matrix Multiply3/1
  Constant1/1 -> Matrix Multiply3/2
  Matrix Multiply3/1 -> Matrix Multiply1/2
  delta_function/1 -> Matrix Multiply1/1
  Matrix Multiply1/1 -> Matrix Multiply2/1
  x/1 -> Matrix Multiply2/2
  Matrix Multiply2/1 -> DeltaAx/1

== system cukModelStateSpace/FDI_Device_2/Alarm_Function/If Action Subsystem ==
  In1 : Inport
  Action Port : ActionPort  ActionPortLabel=if(u1 > 0)
  Out1 : Outport
  wires:
  In1/1 -> Out1/1

== system cukModelStateSpace/FDI_Device_2/Alarm_Function/If Action Subsystem1 ==
  In1 : Inport
  Action Port : ActionPort  ActionPortLabel=else
  Out1 : Outport
  wires:
  In1/1 -> Out1/1

== system cukModelStateSpace/FDI_Device_2/Resiual_Evaluation_Function/If Action Subsystem ==
  r : Inport
  Action Port : ActionPort  ActionPortLabel=if(u1 >= T)
  J : Outport
  wires:
  r/1 -> J/1  "||r1||"

== system cukModelStateSpace/FDI_Device_2/Resiual_Evaluation_Function/If Action Subsystem1 ==
  r : Inport
  Action Port : ActionPort  ActionPortLabel=else
  Norm3 : PhdLibrary/Norms/Norm
      settings: SourceProductName=Phd Diego
  J : Outport
  wires:
  r/1 -> Norm3/1
  Norm3/1 -> J/1  "||r1||"

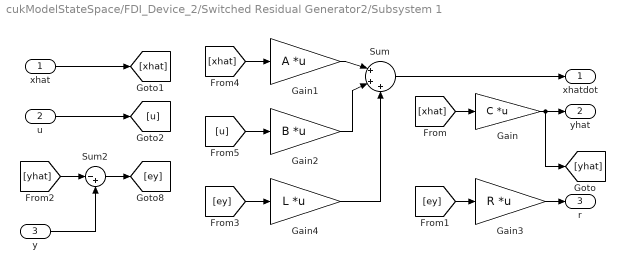
== system cukModelStateSpace/FDI_Device_2/Switched Residual Generator2/Subsystem 1 ==
  xhat : Inport
  u : Inport  Port=2
  y : Inport  Port=3
  Gain : Gain  Gain=C  Multiplication=Matrix(K*u) (u vector)
  Gain1 : Gain  Gain=A  Multiplication=Matrix(K*u) (u vector)
  Gain2 : Gain  Gain=B  Multiplication=Matrix(K*u) (u vector)
  Gain3 : Gain  Gain=R  Multiplication=Matrix(K*u) (u vector)
  Gain4 : Gain  Gain=L  Multiplication=Matrix(K*u) (u vector)
  Sum : Sum  Inputs=|+++
  Sum2 : Sum  Inputs=|-+
  xhatdot : Outport
  yhat : Outport  Port=2
  r : Outport  Port=3
  wires:
  [ey] -> Gain4/1
  Gain4/1 -> Sum/3
  Gain2/1 -> Sum/2
  [u] -> Gain2/1
  Gain1/1 -> Sum/1
  [xhat] -> Gain1/1
  u/1 -> [u]
  Gain3/1 -> r/1
  [ey] -> Gain3/1
  [xhat] -> Gain/1
  xhat/1 -> [xhat]
  Gain/1 -> [yhat], yhat/1
  Sum/1 -> xhatdot/1
  y/1 -> Sum2/2
  [yhat] -> Sum2/1
  Sum2/1 -> [ey]

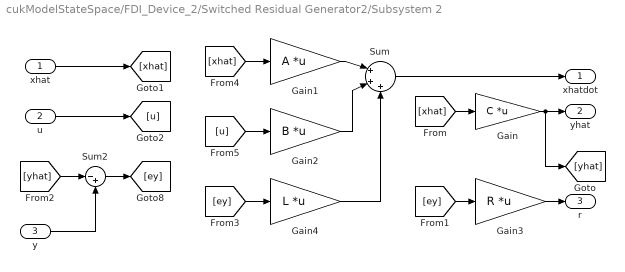
== system cukModelStateSpace/FDI_Device_2/Switched Residual Generator2/Subsystem 2 ==
  xhat : Inport
  u : Inport  Port=2
  y : Inport  Port=3
  Gain : Gain  Gain=C  Multiplication=Matrix(K*u) (u vector)
  Gain1 : Gain  Gain=A  Multiplication=Matrix(K*u) (u vector)
  Gain2 : Gain  Gain=B  Multiplication=Matrix(K*u) (u vector)
  Gain3 : Gain  Gain=R  Multiplication=Matrix(K*u) (u vector)
  Gain4 : Gain  Gain=L  Multiplication=Matrix(K*u) (u vector)
  Sum : Sum  Inputs=|+++
  Sum2 : Sum  Inputs=|-+
  xhatdot : Outport
  yhat : Outport  Port=2
  r : Outport  Port=3
  wires:
  [ey] -> Gain4/1
  Gain4/1 -> Sum/3
  Gain2/1 -> Sum/2
  [u] -> Gain2/1
  Gain1/1 -> Sum/1
  [xhat] -> Gain1/1
  u/1 -> [u]
  Gain3/1 -> r/1
  [ey] -> Gain3/1
  [xhat] -> Gain/1
  xhat/1 -> [xhat]
  Gain/1 -> [yhat], yhat/1
  Sum/1 -> xhatdot/1
  y/1 -> Sum2/2
  [yhat] -> Sum2/1
  Sum2/1 -> [ey]

== system cukModelStateSpace/FDI_Device_3/Alarm_Function/If Action Subsystem ==
  In1 : Inport
  Action Port : ActionPort  ActionPortLabel=if(u1 > 0)
  Out1 : Outport
  wires:
  In1/1 -> Out1/1

== system cukModelStateSpace/FDI_Device_3/Alarm_Function/If Action Subsystem1 ==
  In1 : Inport
  Action Port : ActionPort  ActionPortLabel=else
  Out1 : Outport
  wires:
  In1/1 -> Out1/1

== system cukModelStateSpace/FDI_Device_3/Resiual_Evaluation_Function/If Action Subsystem ==
  r : Inport
  Action Port : ActionPort  ActionPortLabel=if(u1 >= T)
  J : Outport
  wires:
  r/1 -> J/1  "||r1||"

== system cukModelStateSpace/FDI_Device_3/Resiual_Evaluation_Function/If Action Subsystem1 ==
  r : Inport
  Action Port : ActionPort  ActionPortLabel=else
  Norm3 : PhdLibrary/Norms/Norm
      settings: SourceProductName=Phd Diego
  J : Outport
  wires:
  r/1 -> Norm3/1
  Norm3/1 -> J/1  "||r1||"

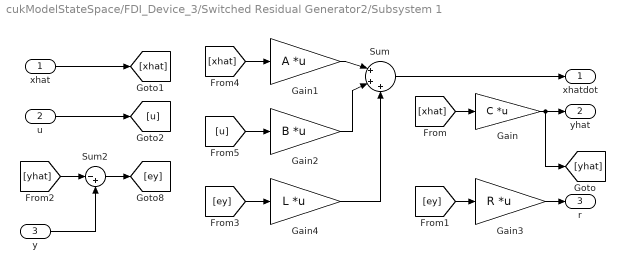
== system cukModelStateSpace/FDI_Device_3/Switched Residual Generator2/Subsystem 1 ==
  xhat : Inport
  u : Inport  Port=2
  y : Inport  Port=3
  Gain : Gain  Gain=C  Multiplication=Matrix(K*u) (u vector)
  Gain1 : Gain  Gain=A  Multiplication=Matrix(K*u) (u vector)
  Gain2 : Gain  Gain=B  Multiplication=Matrix(K*u) (u vector)
  Gain3 : Gain  Gain=R  Multiplication=Matrix(K*u) (u vector)
  Gain4 : Gain  Gain=L  Multiplication=Matrix(K*u) (u vector)
  Sum : Sum  Inputs=|+++
  Sum2 : Sum  Inputs=|-+
  xhatdot : Outport
  yhat : Outport  Port=2
  r : Outport  Port=3
  wires:
  [ey] -> Gain4/1
  Gain4/1 -> Sum/3
  Gain2/1 -> Sum/2
  [u] -> Gain2/1
  Gain1/1 -> Sum/1
  [xhat] -> Gain1/1
  u/1 -> [u]
  Gain3/1 -> r/1
  [ey] -> Gain3/1
  [xhat] -> Gain/1
  xhat/1 -> [xhat]
  Gain/1 -> [yhat], yhat/1
  Sum/1 -> xhatdot/1
  y/1 -> Sum2/2
  [yhat] -> Sum2/1
  Sum2/1 -> [ey]

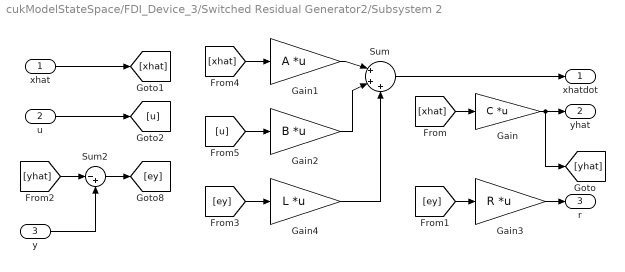
== system cukModelStateSpace/FDI_Device_3/Switched Residual Generator2/Subsystem 2 ==
  xhat : Inport
  u : Inport  Port=2
  y : Inport  Port=3
  Gain : Gain  Gain=C  Multiplication=Matrix(K*u) (u vector)
  Gain1 : Gain  Gain=A  Multiplication=Matrix(K*u) (u vector)
  Gain2 : Gain  Gain=B  Multiplication=Matrix(K*u) (u vector)
  Gain3 : Gain  Gain=R  Multiplication=Matrix(K*u) (u vector)
  Gain4 : Gain  Gain=L  Multiplication=Matrix(K*u) (u vector)
  Sum : Sum  Inputs=|+++
  Sum2 : Sum  Inputs=|-+
  xhatdot : Outport
  yhat : Outport  Port=2
  r : Outport  Port=3
  wires:
  [ey] -> Gain4/1
  Gain4/1 -> Sum/3
  Gain2/1 -> Sum/2
  [u] -> Gain2/1
  Gain1/1 -> Sum/1
  [xhat] -> Gain1/1
  u/1 -> [u]
  Gain3/1 -> r/1
  [ey] -> Gain3/1
  [xhat] -> Gain/1
  xhat/1 -> [xhat]
  Gain/1 -> [yhat], yhat/1
  Sum/1 -> xhatdot/1
  y/1 -> Sum2/2
  [yhat] -> Sum2/1
  Sum2/1 -> [ey]

== system cukModelStateSpace/FDI_Device_4/Alarm_Function/If Action Subsystem ==
  In1 : Inport
  Action Port : ActionPort  ActionPortLabel=if(u1 > 0)
  Out1 : Outport
  wires:
  In1/1 -> Out1/1

== system cukModelStateSpace/FDI_Device_4/Alarm_Function/If Action Subsystem1 ==
  In1 : Inport
  Action Port : ActionPort  ActionPortLabel=else
  Out1 : Outport
  wires:
  In1/1 -> Out1/1

== system cukModelStateSpace/FDI_Device_4/Resiual_Evaluation_Function1/If Action Subsystem ==
  r : Inport
  Action Port : ActionPort
  J : Outport
  wires:
  r/1 -> J/1  "||r1||"

== system cukModelStateSpace/FDI_Device_4/Resiual_Evaluation_Function1/If Action Subsystem1 ==
  r : Inport
  Action Port : ActionPort
  Norm3 : PhdLibrary/Norms/Norm
      settings: SourceProductName=Phd Diego
  J : Outport
  wires:
  r/1 -> Norm3/1
  Norm3/1 -> J/1  "||r1||"

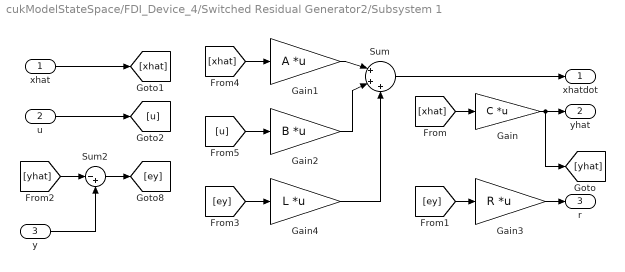
== system cukModelStateSpace/FDI_Device_4/Switched Residual Generator2/Subsystem 1 ==
  xhat : Inport
  u : Inport  Port=2
  y : Inport  Port=3
  Gain : Gain  Gain=C  Multiplication=Matrix(K*u) (u vector)
  Gain1 : Gain  Gain=A  Multiplication=Matrix(K*u) (u vector)
  Gain2 : Gain  Gain=B  Multiplication=Matrix(K*u) (u vector)
  Gain3 : Gain  Gain=R  Multiplication=Matrix(K*u) (u vector)
  Gain4 : Gain  Gain=L  Multiplication=Matrix(K*u) (u vector)
  Sum : Sum  Inputs=|+++
  Sum2 : Sum  Inputs=|-+
  xhatdot : Outport
  yhat : Outport  Port=2
  r : Outport  Port=3
  wires:
  [ey] -> Gain4/1
  Gain4/1 -> Sum/3
  Gain2/1 -> Sum/2
  [u] -> Gain2/1
  Gain1/1 -> Sum/1
  [xhat] -> Gain1/1
  u/1 -> [u]
  Gain3/1 -> r/1
  [ey] -> Gain3/1
  [xhat] -> Gain/1
  xhat/1 -> [xhat]
  Gain/1 -> [yhat], yhat/1
  Sum/1 -> xhatdot/1
  y/1 -> Sum2/2
  [yhat] -> Sum2/1
  Sum2/1 -> [ey]

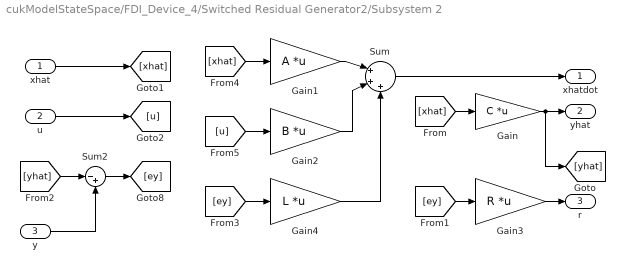
== system cukModelStateSpace/FDI_Device_4/Switched Residual Generator2/Subsystem 2 ==
  xhat : Inport
  u : Inport  Port=2
  y : Inport  Port=3
  Gain : Gain  Gain=C  Multiplication=Matrix(K*u) (u vector)
  Gain1 : Gain  Gain=A  Multiplication=Matrix(K*u) (u vector)
  Gain2 : Gain  Gain=B  Multiplication=Matrix(K*u) (u vector)
  Gain3 : Gain  Gain=R  Multiplication=Matrix(K*u) (u vector)
  Gain4 : Gain  Gain=L  Multiplication=Matrix(K*u) (u vector)
  Sum : Sum  Inputs=|+++
  Sum2 : Sum  Inputs=|-+
  xhatdot : Outport
  yhat : Outport  Port=2
  r : Outport  Port=3
  wires:
  [ey] -> Gain4/1
  Gain4/1 -> Sum/3
  Gain2/1 -> Sum/2
  [u] -> Gain2/1
  Gain1/1 -> Sum/1
  [xhat] -> Gain1/1
  u/1 -> [u]
  Gain3/1 -> r/1
  [ey] -> Gain3/1
  [xhat] -> Gain/1
  xhat/1 -> [xhat]
  Gain/1 -> [yhat], yhat/1
  Sum/1 -> xhatdot/1
  y/1 -> Sum2/2
  [yhat] -> Sum2/1
  Sum2/1 -> [ey]

== system cukModelStateSpace/Sensor_Faults_Generator/Fault_Generation_1/Switch Case Action Subsystem ==
  In1 : Inport
  Action Port : ActionPort  ActionPortLabel=case [ 1 ]:
  Out1 : Outport
  wires:
  In1/1 -> Out1/1

== system cukModelStateSpace/Sensor_Faults_Generator/Fault_Generation_1/Switch Case Action Subsystem1 ==
  In1 : Inport
  Action Port : ActionPort  ActionPortLabel=case [ 2 ]:
  Out1 : Outport
  wires:
  In1/1 -> Out1/1

== system cukModelStateSpace/Sensor_Faults_Generator/Fault_Generation_1/Switch Case Action Subsystem2 ==
  In1 : Inport
  Action Port : ActionPort  ActionPortLabel=default:
  Out1 : Outport
  wires:
  In1/1 -> Out1/1

== system cukModelStateSpace/Sensor_Faults_Generator/Fault_Generation_1/Switch Case Action Subsystem3 ==
  In1 : Inport
  Action Port : ActionPort  ActionPortLabel=case [ 0 ]:
  Out1 : Outport
  wires:
  In1/1 -> Out1/1

== system cukModelStateSpace/Sensor_Faults_Generator/Fault_Generation_2/Switch Case Action Subsystem ==
  In1 : Inport
  Action Port : ActionPort  ActionPortLabel=case [ 1 ]:
  Out1 : Outport
  wires:
  In1/1 -> Out1/1

== system cukModelStateSpace/Sensor_Faults_Generator/Fault_Generation_2/Switch Case Action Subsystem1 ==
  In1 : Inport
  Action Port : ActionPort  ActionPortLabel=case [ 2 ]:
  Out1 : Outport
  wires:
  In1/1 -> Out1/1

== system cukModelStateSpace/Sensor_Faults_Generator/Fault_Generation_2/Switch Case Action Subsystem2 ==
  In1 : Inport
  Action Port : ActionPort  ActionPortLabel=default:
  Out1 : Outport
  wires:
  In1/1 -> Out1/1

== system cukModelStateSpace/Sensor_Faults_Generator/Fault_Generation_2/Switch Case Action Subsystem3 ==
  In1 : Inport
  Action Port : ActionPort  ActionPortLabel=case [ 0 ]:
  Out1 : Outport
  wires:
  In1/1 -> Out1/1

== system cukModelStateSpace/Sensor_Faults_Generator/Fault_Generation_4/Switch Case Action Subsystem ==
  In1 : Inport
  Action Port : ActionPort  ActionPortLabel=case [ 1 ]:
  Out1 : Outport
  wires:
  In1/1 -> Out1/1

== system cukModelStateSpace/Sensor_Faults_Generator/Fault_Generation_4/Switch Case Action Subsystem1 ==
  In1 : Inport
  Action Port : ActionPort  ActionPortLabel=case [ 2 ]:
  Out1 : Outport
  wires:
  In1/1 -> Out1/1

== system cukModelStateSpace/Sensor_Faults_Generator/Fault_Generation_4/Switch Case Action Subsystem2 ==
  In1 : Inport
  Action Port : ActionPort  ActionPortLabel=default:
  Out1 : Outport
  wires:
  In1/1 -> Out1/1

== system cukModelStateSpace/Sensor_Faults_Generator/Fault_Generation_4/Switch Case Action Subsystem3 ==
  In1 : Inport
  Action Port : ActionPort  ActionPortLabel=case [ 0 ]:
  Out1 : Outport
  wires:
  In1/1 -> Out1/1

== system cukModelStateSpace/Uncertain_Cuk/Uncertain Cuk/Subsystem ==
  x : Inport
  u : Inport  Port=2
  Gain : Gain  Gain=B  Multiplication=Matrix(K*u) (u vector)
  Gain1 : Gain  Gain=A  Multiplication=Matrix(K*u) (u vector)
  Gain2 : Gain  Gain=C  Multiplication=Matrix(K*u) (u vector)
  Sum : Sum  Inputs=|++
  xdot : Outport
  y : Outport  Port=2
  wires:
  u/1 -> Gain/1
  x/1 -> Gain2/1, Gain1/1
  Gain1/1 -> Sum/1
  Gain/1 -> Sum/2
  Sum/1 -> xdot/1
  Gain2/1 -> y/1

== system cukModelStateSpace/Uncertain_Cuk/Uncertain Cuk/Subsystem1 ==
  x : Inport
  u : Inport  Port=2
  Gain : Gain  Gain=B  Multiplication=Matrix(K*u) (u vector)
  Gain1 : Gain  Gain=A  Multiplication=Matrix(K*u) (u vector)
  Gain2 : Gain  Gain=C  Multiplication=Matrix(K*u) (u vector)
  Sum : Sum  Inputs=|++
  xdot : Outport
  y : Outport  Port=2
  wires:
  u/1 -> Gain/1
  x/1 -> Gain2/1, Gain1/1
  Gain1/1 -> Sum/1
  Gain/1 -> Sum/2
  Sum/1 -> xdot/1
  Gain2/1 -> y/1
